simulink model "CollisionAvoidance"  (Simulink 8.5)
settings: Solver=FixedStepDiscrete  StartTime=0.0  StopTime=10.0  RelTol=1e-3
libraries: simulink x3
settings Model: Creator=gwilli10  LastModifiedBy=jonah  CovSFcnEnable=off
settings DataIOCC: SignalLoggingSaveFormat=Dataset
settings OptimizationCC: ExpressionDepthLimit=128  OptimizeModelRefInitCode=on  LifeSpan=1
settings DebuggingCC: UnderspecifiedInitializationDetection=Simplified  MergeDetectMultiDrivingBlocksExec=error  SolverPrmCheckMsg=warning  FcnCallInpInsideContextMsg=EnableAllAsError  StateNameClashWarn=none
settings HardwareCC: ProdIntDivRoundTo=Floor  ProdEndianess=LittleEndian  ProdHWDeviceType=Generic->32-bit Embedded Processor
settings RTWCC: SystemTargetFile=ert.tlc  GenCodeOnly=on  TemplateMakefile=ert_default_tmf  Description=Embedded Coder
settings CodeAppCC: IgnoreCustomStorageClasses=off  MATLABSourceComments=on
settings ERTTargetCC: MultiwordLength=2048  GenerateSampleERTMain=on  MultiInstanceERTCode=on  CodeInterfacePackaging=Reusable function  RootIOFormat=Structure reference  ERTCustomFileTemplate=example_file_process.tlc  ERTFilePackagingFormat=CompactWithDataFile  SuppressUnreachableDefaultCases=off

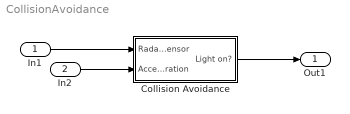
== system CollisionAvoidance ==
  In1 : Inport  OutDataTypeStr=single
  In2 : Inport  Port=2  OutDataTypeStr=single
  "Collision Avoidance " : Subsystem
  Out1 : Outport
  wires:
  In1/1 -> "Collision Avoidance "/1(Radar sensor)
  In2/1 -> "Collision Avoidance "/2(Acceleration)
  "Collision Avoidance "/1(Light on?) -> Out1/1

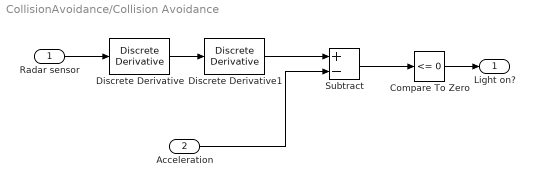
== system CollisionAvoidance/Collision Avoidance  ==
  Radar sensor : Inport
  Acceleration : Inport  Port=2
  Compare To Zero : simulink/Logic and Bit Operations/Compare To Zero  relop=<=  OutDataTypeStr=boolean
  Discrete Derivative : simulink/Discrete/Discrete Derivative  gainval=1.0  ICPrevScaledInput=0.0  InputProcessing=Inherited  OutMin=[]  OutMax=[]  OutDataType=fixdt(1, 16)  OutScaling=2^-10  DoSatur=off
  Discrete Derivative1 : simulink/Discrete/Discrete Derivative  gainval=1.0  ICPrevScaledInput=0.0  InputProcessing=Inherited  OutMin=[]  OutMax=[]  OutDataType=fixdt(1, 16)  OutScaling=2^-10  DoSatur=off
  Subtract : Sum  Inputs=+-
  Light on? : Outport
  wires:
  Acceleration/1 -> Subtract/2
  Subtract/1 -> Compare To Zero/1
  Compare To Zero/1 -> Light on?/1
  Radar sensor/1 -> Discrete Derivative/1
  Discrete Derivative/1 -> Discrete Derivative1/1
  Discrete Derivative1/1 -> Subtract/1
